simulink library "speedgoatlib_IO682"  (R2024b)
settings: Solver=FixedStepAuto  StartTime=0.0  StopTime=10.0  RelTol=1e-3  EnableMultiTasking=on
undefined symbols (not defined in the file): sg_io682_receive_m_v4, sg_io682_send_m_v4, sg_io682_setup_m_v4, sg_io682_update_scheduled_messages_m_v4, sgarinc429
settings Model: Creator=cschafft  LastModifiedBy=speedgoat\jenkins
settings SolverCC: ConcurrentTasks=on  AlgebraicLoopSolver=TrustRegion  AutoInsertRateTranBlk=on  InsertRTBMode=Never (minimum delay)
settings DataIOCC: LimitDataPoints=on  SaveFormat=StructureWithTime  ReturnWorkspaceOutputs=off
settings OptimizationCC: BlockReduction=off  OptimizeBlockIOStorage=off  BufferReuse=off  ReuseModelBlockBuffer=off  GlobalBufferReuse=off  ExpressionFolding=off  LocalBlockOutputs=off  OptimizeDataStoreBuffers=off  BusAssignmentInplaceUpdate=off
settings DebuggingCC: UnconnectedInputMsg=warning  UnconnectedOutputMsg=warning  UnconnectedLineMsg=warning  AllowSymbolicDim=off  SFUnexpectedBacktrackingDiag=warning  SFNoUnconditionalDefaultTransitionDiag=warning  SFExecutionAtInitializationDiag=none  ArithmeticOperatorsInVariantConditions=warning
settings HardwareCC: ProdBitPerPointer=32  ProdBitPerSizeT=32  ProdBitPerPtrDiffT=32  ProdLargestAtomicFloat=None  ProdWordSize=32  ProdLongLongMode=on  ProdHWDeviceType=Generic->32-bit x86 compatible
settings ModelReferenceCC: EnableRefExpFcnMdlSchedulingChecks=on  PropagateSignalLabelsOutOfModel=off
settings SFSimCC: SimUseLocalCustomCode=off  CustomCodeUndefinedFunction=UseInterfaceOnly
settings RTWCC: Description=Simulink Real-Time  SystemTargetFile=slrt.tlc  TemplateMakefile=slrt_default_tmf  RTWUseLocalCustomCode=off  RTWCompilerOptimization=on  GPUComputeCapability=3.5  DLArmComputeVersion=19.05
settings CodeAppCC: StateflowObjectComments=on
settings SimulinkRealTimeCC: SubcomponentCodeInterfacePackaging=Reusable function  SupportVariableSizeSignals=on  InstructionSetFMA=off  OptimizeReductions=off  LogToMDFFile=off  RL32LogTETModifier=off
settings ConfigComp: CovMetricSettings=dw  CovSaveCumulativeToWorkspaceVar=on  CovSaveSingleToWorkspaceVar=on  CovExternalEMLEnable=off  CovBoundaryAbsTol=1.0e-5

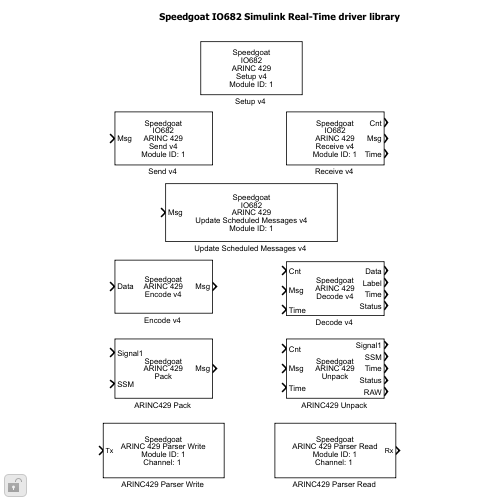
[thumbnail: Simulink's stored preview of the top-level diagram]
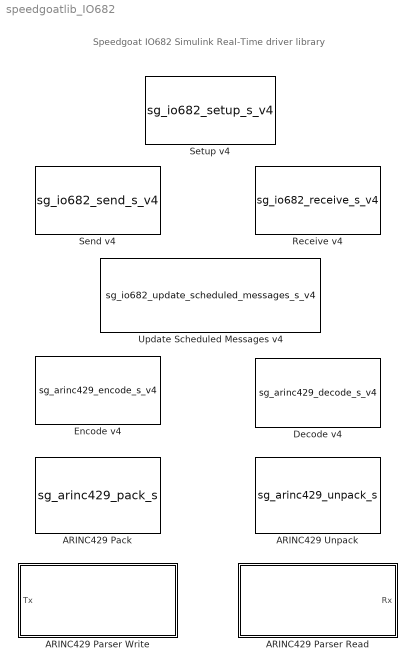
== system speedgoatlib_IO682 ==
  note: Speedgoat IO682 Simulink Real-Time driver library
  "ARINC429 Pack " : S-Function  LoadFcn=sgarinc429.LoadFcnPackUnpack();  FunctionName=sg_arinc429_pack_s  Parameters=sFunParams.decLabel,parSdi,parSsm,sFunParams.signals,sFunParams.hasSsmSig  SFunctionDeploymentMode=off  EnableBusSupport=off  mask(pack_arinc429){parLabel=102, parSdi=0, parSsm=3, parSignals={'Signal1','11','16','BNR','256','0.01','0','-Inf','Inf','off';'SSM','30','2','SSM','1','1','0','-Inf','Inf','off'}}
      mask prompts: parLabel "Label"; parSdi "SDI"; parSsm "SSM"; parSignals "Signals"
      mask help: Speedgoat Driver Block<br>ARINC 429 - Pack<br><br>&copy; 2007 - 2026, Speedgoat GmbH, <a href="matlab: web('www.speedgoat.com','-browser');">www.speedgoat.com</a>
      mask init:
      | sFunParams = sg_arinc429_pack_m.maskInitialization();
      mask Help: eval('sg.utils.help.show(''io_main/refentry_arinc429_pack'');')
      mask DialogControl btnAddSig Prompt: Add Signal
      mask DialogControl btnAddSig Callback: sg_arinc429_pack_m.addSigBtnClb();
      mask DialogControl btnDelSig Prompt: Delete Signal
      mask DialogControl btnDelSig Callback: sg_arinc429_pack_m.delSigBtnClb();
      mask Display: disp('Speedgoat\nARINC 429\nPack');port_label('output',1,'Msg');port_label('input',1,'Signal1');port_label('input',2,'SSM');
  "ARINC429 Parser Read " : Subsystem  mask(read_parser_arinc429){}
      settings: OpenFcn=sgarinc429.OpenFcnRead();
      mask Help: eval('sg.utils.help.show(''io_main/refentry_arinc429_parser_read'');')
      mask Display: disp('Speedgoat\nARINC 429 Parser Read\nModule ID: 1\nChannel: 1 ');
  "ARINC429 Parser Write " : Subsystem  mask(write_parser_arinc429){}
      settings: OpenFcn=sgarinc429.OpenFcnWrite();
      mask Help: eval('sg.utils.help.show(''io_main/refentry_arinc429_parser_write'');')
      mask Display: disp('Speedgoat\nARINC 429 Parser Write\nModule ID: 1\nChannel: 1 ');
  "ARINC429 Unpack " : S-Function  LoadFcn=sgarinc429.LoadFcnPackUnpack();  FunctionName=sg_arinc429_unpack_s  Parameters=sFunParams.decLabel,parSdi,parEnTimeTag,parEnStatus,parEnRaw,sFunParams.signals,sFunParams.hasSsmSig  SFunctionDeploymentMode=off  EnableBusSupport=off  mask(unpack_arinc429){parLabel=102, parSdi=0, parSignals={'Signal1','11','16','BNR','256','0.01','0','-Inf','Inf','off';'SSM','30','2','SSM','1','1','0','-Inf','Inf','off'}, parEnTimeTag=on, parEnStatus=on, parEnRaw=on}
      mask prompts: parLabel "Label"; parSdi "SDI"; parSignals "Signals"; parEnTimeTag "Enable Timestamp Output"; parEnStatus "Enable Status Output"; parEnRaw "Enable RAW Output"
      mask help: Speedgoat Driver Block<br>ARINC 429 - Unpack<br><br>&copy; 2007 - 2026, Speedgoat GmbH, <a href="matlab: web('www.speedgoat.com','-browser');">www.speedgoat.com</a>
      mask init:
      | sFunParams = sg_arinc429_unpack_m.maskInitialization();
      mask Help: eval('sg.utils.help.show(''io_main/refentry_arinc429_unpack'');')
      mask DialogControl btnAddSig Prompt: Add Signal
      mask DialogControl btnAddSig Callback: sg_arinc429_unpack_m.addSigBtnClb();
      mask DialogControl btnDelSig Prompt: Delete Signal
      mask DialogControl btnDelSig Callback: sg_arinc429_unpack_m.delSigBtnClb();
      mask DialogControl Container3 Prompt: Output Ports
      mask Display: disp('Speedgoat\nARINC 429\nUnpack');port_label('input',1,'Cnt');port_label('input',2,'Msg');port_label('input',3,'Time');port_label('output',1,'Signal1');port_label('output',2,'SSM');port_label('output',3,'Time');port_label('output',4,'Status');port_label('output',5,'RAW');
  "Decode v4 " : S-Function  FunctionName=sg_arinc429_decode_s_v4  Parameters=sFunParams.decLabel, sFunParams.dataType, sFunParams.resolution, sFunParams.sdi, parEnSDIBits, parTimeTags, parHoldLastVal, parStatus, parLabelOutput, parSSMOutput  SFunctionDeploymentMode=off  EnableBusSupport=off  mask(decode_arinc429_v4){parLabel=[002], parDataType=BNR, parResolution=[10], parSdi=[0], parEnSDIBits=off, parHoldLastVal=on, parLabelOutput=on, parSSMOutput=off, parTimeTags=on, parStatus=on}
      mask prompts: parLabel "Label (Octal)"; parDataType "Data Type"; parResolution "Scale"; parSdi "SDI"; parEnSDIBits "Use SDI Bits for Data"; parHoldLastVal "Hold Last Value"; parLabelOutput "Enable Label Output"; parSSMOutput "Enable SSM Output"; parTimeTags "Enable Timestamp Output"; parStatus "Enable Status Output"
      mask help: Speedgoat Driver Block<br>ARINC 429 - Decode<br><br>&copy; 2007 - 2026, Speedgoat GmbH, <a href="matlab: web('www.speedgoat.com','-browser');">www.speedgoat.com</a>
      mask init:
      | sFunParams = sg_arinc429_decode_m_v4.runInitializationCommand();
      mask Help: eval('sg.utils.help.show(''io_main/refentry_arinc429_decode_v4'');')
      mask TypeOptions parDataType: RAW | BNR | BCD | Discretes
      mask Callback parDataType: sg_arinc429_decode_m_v4.dataTypeCallback();
      mask Callback parEnSDIBits: sg_arinc429_decode_m_v4.enableSDIBitsCallback();
      mask Display: disp('Speedgoat\nARINC 429\nDecode v4');port_label('input',1,'Cnt');port_label('input',2,'Msg');port_label('input',3,'Time');port_label('output',1,'Data');port_label('output',2,'Label');port_label('output',3,'Time');port_label('output',4,'Status');
  "Encode v4 " : S-Function  FunctionName=sg_arinc429_encode_s_v4  Parameters=sFunParams.decLabel, sFunParams.dataType, sFunParams.resolution, sFunParams.bits, sFunParams.sdi, sFunParams.ssm, parEnSSM, parEnSDIBits  SFunctionDeploymentMode=off  EnableBusSupport=off  mask(encode_arinc429_v4){parLabel=[002], parDataType=BNR, parResolution=[10], parBits=[19], parSdi=[0], parSsm=[3], parEnSDIBits=off, parEnSSM=off}
      mask prompts: parLabel "Label (Octal)"; parDataType "Data Type"; parResolution "Scale"; parBits "Bits to Send"; parSdi "SDI"; parSsm "SSM"; parEnSDIBits "Use SDI Bits for Data"; parEnSSM "Enable SSM Input"
      mask help: Speedgoat Driver Block<br>ARINC 429 - Encode<br><br>&copy; 2007 - 2026, Speedgoat GmbH, <a href="matlab: web('www.speedgoat.com','-browser');">www.speedgoat.com</a>
      mask init:
      | sFunParams = sg_arinc429_encode_m_v4.runInitializationCommand();
      mask Help: eval('sg.utils.help.show(''io_main/refentry_arinc429_encode_v4'');')
      mask TypeOptions parDataType: RAW | BNR | BCD | Discretes
      mask Callback parDataType: sg_arinc429_encode_m_v4.dataTypeCallback();
      mask Callback parEnSDIBits: sg_arinc429_encode_m_v4.enableSDIBitsCallback();
      mask Callback parEnSSM: sg_arinc429_encode_m_v4.enableSSMCallback();
      mask Display: disp('Speedgoat\nARINC 429\nEncode v4');port_label('output',1,'Msg');port_label('input',1,'Data');
  "Receive v4 " : S-Function  InitFcn=sg_io682_receive_m_v4.runInitFcn();  FunctionName=sg_io682_receive_s_v4  Parameters=parModuleId, parChannel, parMaxWords, parSampleTime, parEnTimeTags  SFunctionDeploymentMode=off  EnableBusSupport=off  mask(receive_IO682_v4){parModuleId=1, parChannel=1, parMaxWords=50, parSampleTime=-1, parEnTimeTags=on}
      mask prompts: parModuleId "Module ID"; parChannel "Channel"; parMaxWords "Max Number of Messages to Return"; parSampleTime "Sample Time [s]"; parEnTimeTags "Provide Timestamps"
      mask help: Speedgoat Driver Block<br>IO682 - Receive<br><br>&copy; 2007 - 2026, Speedgoat GmbH, <a href="matlab: web('www.speedgoat.com','-browser');">www.speedgoat.com</a>
      mask init:
      | sg_io682_receive_m_v4.runMaskInitialization();
      mask Help: eval('sg.utils.help.show(''io_main/refentry_io682_receive_v4'');')
      mask TypeOptions parChannel: 1 | 2 | 3 | 4 | 5 | 6 | 7 | 8 | 9 | 10 | 11 | 12 | 13 | 14 | 15 | 16
      mask Display: disp('Speedgoat\nIO682\nARINC 429\nReceive v4\nModule ID: 1');port_label('output',1,'Cnt');port_label('output',2,'Msg');port_label('output',3,'Time');
  "Send v4 " : S-Function  InitFcn=sg_io682_send_m_v4.runInitFcn();  FunctionName=sg_io682_send_s_v4  Parameters=parModuleId, parChannel, parSampleTime, parTxCtrl  SFunctionDeploymentMode=off  EnableBusSupport=off  mask(send_IO682_v4){parModuleId=1, parChannel=1, parSampleTime=-1, parTxCtrl=off}
      mask prompts: parModuleId "Module ID"; parChannel "Channel"; parSampleTime "Sample Time [s]"; parTxCtrl "Show Transmission Control Input"
      mask help: Speedgoat Driver Block<br>IO682 - Send<br><br>&copy; 2007 - 2026, Speedgoat GmbH, <a href="matlab: web('www.speedgoat.com','-browser');">www.speedgoat.com</a>
      mask init:
      | sg_io682_send_m_v4.runMaskInitialization();
      mask Help: eval('sg.utils.help.show(''io_main/refentry_io682_send_v4'');')
      mask TypeOptions parChannel: 1 | 2 | 3 | 4 | 5 | 6 | 7 | 8 | 9 | 10 | 11 | 12 | 13 | 14 | 15 | 16
      mask Display: disp('Speedgoat\nIO682\nARINC 429\nSend v4\nModule ID: 1');port_label('input',1,'Msg');
  "Setup v4 " : S-Function  InitFcn=sg_io682_setup_m_v4.runInitFcn();  FunctionName=sg_io682_setup_s_v4  Parameters=parModuleId, parBoardVariant, parPciSlot, parHwDeviceId, parScheduledMessages, parChInConfig,parChOutConfig  SFunctionModules=sg_io682_v4  SFunctionDeploymentMode=off  EnableBusSupport=off  mask(setup_IO682_v4){parModuleId=1, parBoardVariant=IO682-2-2, parPciSlot=-1, parChannelMode=Manual, parInBitRate1=100000, parInBufferMode1=Individual, parInEnable1=on, parInParity1=on, parInInternalWrap1=off, parInBitRate2=100000, parInBufferMode2=Individual, parInEnable2=on, parInParity2=on, parInInternalWrap2=off, parInBitRate3=100000, parInBufferMode3=Individual, parInEnable3=on, parInParity3=on, parInInternalWrap3=off, parInBitRate4=100000, parInBufferMode4=Individual, parInEnable4=on, parInParity4=on, parInInternalWrap4=off, parInBitRate5=100000, parInBufferMode5=Individual, parInEnable5=on, parInParity5=on, parInInternalWrap5=off, parInBitRate6=100000, parInBufferMode6=Individual, parInEnable6=on, parInParity6=on, parInInternalWrap6=off, parInBitRate7=100000, parInBufferMode7=Individual, parInEnable7=on, parInParity7=on, parInInternalWrap7=off, parInBitRate8=100000, parInBufferMode8=Individual, parInEnable8=on, parInParity8=on, parInInternalWrap8=off, parInBitRate9=100000, parInBufferMode9=Individual, parInEnable9=on, parInParity9=on, parInInternalWrap9=off, parInBitRate10=100000, parInBufferMode10=Individual, parInEnable10=on, parInParity10=on, parInInternalWrap10=off, parInBitRate11=100000, parInBufferMode11=Individual, parInEnable11=on, parInParity11=on, parInInternalWrap11=off, parInBitRate12=100000, parInBufferMode12=Individual, parInEnable12=on, parInParity12=on, parInInternalWrap12=off, parInBitRate13=100000, parInBufferMode13=Individual, parInEnable13=on, parInParity13=on, parInInternalWrap13=off, parInBitRate14=100000, parInBufferMode14=Individual, parInEnable14=on, parInParity14=on, parInInternalWrap14=off, parInBitRate15=100000, parInBufferMode15=Individual, parInEnable15=on, parInParity15=on, parInInternalWrap15=off, parInBitRate16=100000, parInBufferMode16=Individual, parInEnable16=on, parInParity16=on, parInInternalWrap16=off, parOutBitRate1=100000, parOutParity1=Odd, parOutProtocolError1=None, parOutEnable1=on, parOutBitRate2=100000, parOutParity2=Odd, parOutProtocolError2=None, parOutEnable2=on, parOutBitRate3=100000, parOutParity3=Odd, parOutProtocolError3=None, parOutEnable3=on, parOutBitRate4=100000, parOutParity4=Odd, parOutProtocolError4=None, parOutEnable4=on, parOutBitRate5=100000, parOutParity5=Odd, parOutProtocolError5=None, parOutEnable5=on, parOutBitRate6=100000, parOutParity6=Odd, parOutProtocolError6=None, parOutEnable6=on, parOutBitRate7=100000, parOutParity7=Odd, parOutProtocolError7=None, parOutEnable7=on, parOutBitRate8=100000, parOutParity8=Odd, parOutProtocolError8=None, parOutEnable8=on, parOutBitRate9=100000, parOutParity9=Odd, parOutProtocolError9=None, parOutEnable9=on, parOutBitRate10=100000, parOutParity10=Odd, parOutProtocolError10=None, parOutEnable10=on, parOutBitRate11=100000, parOutParity11=Odd, parOutProtocolError11=None, parOutEnable11=on, parOutBitRate12=100000, parOutParity12=Odd, parOutProtocolError12=None, parOutEnable12=on, parOutBitRate13=100000, parOutParity13=Odd, parOutProtocolError13=None, parOutEnable13=on, parOutBitRate14=100000, parOutParity14=Odd, parOutProtocolError14=None, parOutEnable14=on, parOutBitRate15=100000, parOutParity15=Odd, parOutProtocolError15=None, parOutEnable15=on, parOutBitRate16=100000, parOutParity16=Odd, parOutProtocolError16=None, parOutEnable16=on, parChConfigFile='', parScheduleMode=Manual, parScheduledMsgConfigFile='', parHwDeviceId=hex2dec('0830'), parChInConfig=[158 8 7 7 1;158 8 7 7 1], parChOutConfig=[158 0 4 7;158 0 4 7], parScheduledMessages=0}
      mask prompts: parModuleId "Module ID"; parBoardVariant "IO682 Variant"; parPciSlot "PCI Slot (-1: autosearch)"; parChannelMode "Mode"; parInBitRate1 "Bit Rate"; parInBufferMode1 "Buffer Mode"; parInEnable1 "Enable"; parInParity1 "Parity Check"; parInInternalWrap1 "Internal Wrap"; parInBitRate2 "Bit Rate"; parInBufferMode2 "Buffer Mode"; parInEnable2 "Enable"; parInParity2 "Parity Check"; parInInternalWrap2 "Internal Wrap"; parInBitRate3 "Bit Rate"; parInBufferMode3 "Buffer Mode"; parInEnable3 "Enable"; parInParity3 "Parity Check"; parInInternalWrap3 "Internal Wrap"; parInBitRate4 "Bit Rate"; parInBufferMode4 "Buffer Mode"; parInEnable4 "Enable"; parInParity4 "Parity Check"; parInInternalWrap4 "Internal Wrap"; parInBitRate5 "Bit Rate"; parInBufferMode5 "Buffer Mode"; parInEnable5 "Enable"; parInParity5 "Parity Check"; parInInternalWrap5 "Internal Wrap"; parInBitRate6 "Bit Rate"; parInBufferMode6 "Buffer Mode"; parInEnable6 "Enable"; parInParity6 "Parity Check"; parInInternalWrap6 "Internal Wrap"; parInBitRate7 "Bit Rate"; parInBufferMode7 "Buffer Mode"; parInEnable7 "Enable"; parInParity7 "Parity Check"; parInInternalWrap7 "Internal Wrap"; parInBitRate8 "Bit Rate"; parInBufferMode8 "Buffer Mode"; parInEnable8 "Enable"; parInParity8 "Parity Check"; parInInternalWrap8 "Internal Wrap"; parInBitRate9 "Bit Rate"; parInBufferMode9 "Buffer Mode"; parInEnable9 "Enable"; parInParity9 "Parity Check"; parInInternalWrap9 "Internal Wrap"; parInBitRate10 "Bit Rate"; parInBufferMode10 "Buffer Mode"; parInEnable10 "Enable"; parInParity10 "Parity Check"; parInInternalWrap10 "Internal Wrap"; parInBitRate11 "Bit Rate"; parInBufferMode11 "Buffer Mode"; parInEnable11 "Enable"; parInParity11 "Parity Check"; parInInternalWrap11 "Internal Wrap"; parInBitRate12 "Bit Rate"; parInBufferMode12 "Buffer Mode"; parInEnable12 "Enable"; parInParity12 "Parity Check"; parInInternalWrap12 "Internal Wrap"; parInBitRate13 "Bit Rate"; parInBufferMode13 "Buffer Mode"; parInEnable13 "Enable"; parInParity13 "Parity Check"; parInInternalWrap13 "Internal Wrap"; parInBitRate14 "Bit Rate"; parInBufferMode14 "Buffer Mode"; parInEnable14 "Enable"; parInParity14 "Parity Check"; parInInternalWrap14 "Internal Wrap"; parInBitRate15 "Bit Rate"; parInBufferMode15 "Buffer Mode"; parInEnable15 "Enable"; parInParity15 "Parity Check"; parInInternalWrap15 "Internal Wrap"; parInBitRate16 "Bit Rate"; parInBufferMode16 "Buffer Mode"; parInEnable16 "Enable"; parInParity16 "Parity Check"; parInInternalWrap16 "Internal Wrap"; parOutBitRate1 "Bit Rate"; parOutParity1 "Parity"; parOutProtocolError1 "Protocol Error"; parOutEnable1 "Enable"; parOutBitRate2 "Bit Rate"; parOutParity2 "Parity"; parOutProtocolError2 "Protocol Error"; parOutEnable2 "Enable"; parOutBitRate3 "Bit Rate"; parOutParity3 "Parity"; parOutProtocolError3 "Protocol Error"; parOutEnable3 "Enable"; parOutBitRate4 "Bit Rate"; parOutParity4 "Parity"; parOutProtocolError4 "Protocol Error"; parOutEnable4 "Enable"; parOutBitRate5 "Bit Rate"; parOutParity5 "Parity"; parOutProtocolError5 "Protocol Error"; parOutEnable5 "Enable"; parOutBitRate6 "Bit Rate"; parOutParity6 "Parity"; parOutProtocolError6 "Protocol Error"; parOutEnable6 "Enable"; parOutBitRate7 "Bit Rate"; parOutParity7 "Parity"; parOutProtocolError7 "Protocol Error"; parOutEnable7 "Enable"; parOutBitRate8 "Bit Rate"; parOutParity8 "Parity"; parOutProtocolError8 "Protocol Error"; parOutEnable8 "Enable"; parOutBitRate9 "Bit Rate"; parOutParity9 "Parity"; parOutProtocolError9 "Protocol Error"; parOutEnable9 "Enable"; parOutBitRate10 "Bit Rate"; parOutParity10 "Parity"; parOutProtocolError10 "Protocol Error"; parOutEnable10 "Enable"; parOutBitRate11 "Bit Rate"; parOutParity11 "Parity"; parOutProtocolError11 "Protocol Error"; parOutEnable11 "Enable"; parOutBitRate12 "Bit Rate"; parOutParity12 "Parity"; parOutProtocolError12 "Protocol Error"; parOutEnable12 "Enable"; parOutBitRate13 "Bit Rate"; parOutParity13 "Parity"; parOutProtocolError13 "Protocol Error"; parOutEnable13 "Enable"; parOutBitRate14 "Bit Rate"; parOutParity14 "Parity"; parOutProtocolError14 "Protocol Error"; parOutEnable14 "Enable"; parOutBitRate15 "Bit Rate"; parOutParity15 "Parity"; parOutProtocolError15 "Protocol Error"; parOutEnable15 "Enable"; parOutBitRate16 "Bit Rate"; parOutParity16 "Parity"; parOutProtocolError16 "Protocol Error"; parOutEnable16 "Enable"; parChConfigFile "Channels Configuration File"; parScheduleMode "Mode"; parScheduledMsgConfigFile "Scheduled Messages Configuration File"; parChInConfig "In Ch Config List"; parChOutConfig "Out Ch Config List"; parScheduledMessages "Message List"
      mask help: Speedgoat Driver Block<br>IO682 - Setup<br><br>&copy; 2007 - 2026, Speedgoat GmbH, <a href="matlab: web('www.speedgoat.com','-browser');">www.speedgoat.com</a>
      mask init:
      | sg_io682_setup_m_v4.runMaskInitialization();
      mask Help: eval('sg.utils.help.show(''io_main/refentry_io682_setup_v4'');')
      mask TypeOptions parBoardVariant: IO682-2-2 | IO682-4-4 | IO682-8-8 | IO682-16-16
      mask Callback parBoardVariant: sg_io682_setup_m_v4.runBoardVariantCb();
      mask TypeOptions parChannelMode: Manual | Configuration File
      mask Callback parChannelMode: sg_io682_setup_m_v4.runChannelModeCb();
      mask TypeOptions parInBufferMode1: Individual | Merged
      mask TypeOptions parInBufferMode2: Individual | Merged
      mask TypeOptions parInBufferMode3: Individual | Merged
      mask TypeOptions parInBufferMode4: Individual | Merged
      mask TypeOptions parInBufferMode5: Individual | Merged
      mask TypeOptions parInBufferMode6: Individual | Merged
      mask TypeOptions parInBufferMode7: Individual | Merged
      mask TypeOptions parInBufferMode8: Individual | Merged
      mask TypeOptions parInBufferMode9: Individual | Merged
      mask TypeOptions parInBufferMode10: Individual | Merged
      mask TypeOptions parInBufferMode11: Individual | Merged
      mask TypeOptions parInBufferMode12: Individual | Merged
      mask TypeOptions parInBufferMode13: Individual | Merged
      mask TypeOptions parInBufferMode14: Individual | Merged
      mask TypeOptions parInBufferMode15: Individual | Merged
      mask TypeOptions parInBufferMode16: Individual | Merged
      mask TypeOptions parOutParity1: None | Odd | Even
      mask TypeOptions parOutProtocolError1: None | Bit Count High | Bit Count Low | Short Gap
      mask TypeOptions parOutParity2: None | Odd | Even
      mask TypeOptions parOutProtocolError2: None | Bit Count High | Bit Count Low | Short Gap
      mask TypeOptions parOutParity3: None | Odd | Even
      mask TypeOptions parOutProtocolError3: None | Bit Count High | Bit Count Low | Short Gap
      mask TypeOptions parOutParity4: None | Odd | Even
      mask TypeOptions parOutProtocolError4: None | Bit Count High | Bit Count Low | Short Gap
      mask TypeOptions parOutParity5: None | Odd | Even
      mask TypeOptions parOutProtocolError5: None | Bit Count High | Bit Count Low | Short Gap
      mask TypeOptions parOutParity6: None | Odd | Even
      mask TypeOptions parOutProtocolError6: None | Bit Count High | Bit Count Low | Short Gap
      mask TypeOptions parOutParity7: None | Odd | Even
      mask TypeOptions parOutProtocolError7: None | Bit Count High | Bit Count Low | Short Gap
      mask TypeOptions parOutParity8: None | Odd | Even
      mask TypeOptions parOutProtocolError8: None | Bit Count High | Bit Count Low | Short Gap
      mask TypeOptions parOutParity9: None | Odd | Even
      mask TypeOptions parOutProtocolError9: None | Bit Count High | Bit Count Low | Short Gap
      mask TypeOptions parOutParity10: None | Odd | Even
      mask TypeOptions parOutProtocolError10: None | Bit Count High | Bit Count Low | Short Gap
      mask TypeOptions parOutParity11: None | Odd | Even
      mask TypeOptions parOutProtocolError11: None | Bit Count High | Bit Count Low | Short Gap
      mask TypeOptions parOutParity12: None | Odd | Even
      mask TypeOptions parOutProtocolError12: None | Bit Count High | Bit Count Low | Short Gap
      mask TypeOptions parOutParity13: None | Odd | Even
      mask TypeOptions parOutProtocolError13: None | Bit Count High | Bit Count Low | Short Gap
      mask TypeOptions parOutParity14: None | Odd | Even
      mask TypeOptions parOutProtocolError14: None | Bit Count High | Bit Count Low | Short Gap
      mask TypeOptions parOutParity15: None | Odd | Even
      mask TypeOptions parOutProtocolError15: None | Bit Count High | Bit Count Low | Short Gap
      mask TypeOptions parOutParity16: None | Odd | Even
      mask TypeOptions parOutProtocolError16: None | Bit Count High | Bit Count Low | Short Gap
      mask TypeOptions parScheduleMode: Manual | Configuration File
      mask Callback parScheduleMode: sg_io682_setup_m_v4.runScheduleModeCb();
      mask DialogControl tabMain Prompt: Main
      mask DialogControl boxModuleSettings Prompt: Module Settings
      mask DialogControl tabChannelConfig Prompt: Channel Configuration
      mask DialogControl boxInputChannelConfig Prompt: Input Channels
      mask DialogControl parInChannel1 Prompt: Channel 01:
      mask DialogControl parInChannel2 Prompt: Channel 02:
      mask DialogControl parInChannel3 Prompt: Channel 03:
      mask DialogControl parInChannel4 Prompt: Channel 04:
      mask DialogControl parInChannel5 Prompt: Channel 05:
      mask DialogControl parInChannel6 Prompt: Channel 06:
      mask DialogControl parInChannel7 Prompt: Channel 07:
      mask DialogControl parInChannel8 Prompt: Channel 08:
      mask DialogControl parInChannel9 Prompt: Channel 09:
      mask DialogControl parInChannel10 Prompt: Channel 10:
      mask DialogControl parInChannel11 Prompt: Channel 11:
      mask DialogControl parInChannel12 Prompt: Channel 12:
      mask DialogControl parInChannel13 Prompt: Channel 13:
      mask DialogControl parInChannel14 Prompt: Channel 14:
      mask DialogControl parInChannel15 Prompt: Channel 15:
      mask DialogControl parInChannel16 Prompt: Channel 16:
      mask DialogControl boxOutputChannelConfig Prompt: Output Channels
      mask DialogControl parOutChannel1 Prompt: Channel 01:
      mask DialogControl parOutChannel2 Prompt: Channel 02:
      mask DialogControl parOutChannel3 Prompt: Channel 03:
      mask DialogControl parOutChannel4 Prompt: Channel 04:
      mask DialogControl parOutChannel5 Prompt: Channel 05:
      mask DialogControl parOutChannel6 Prompt: Channel 06:
      mask DialogControl parOutChannel7 Prompt: Channel 07:
      mask DialogControl parOutChannel8 Prompt: Channel 08:
      mask DialogControl parOutChannel9 Prompt: Channel 09:
      mask DialogControl parOutChannel10 Prompt: Channel 10:
      mask DialogControl parOutChannel11 Prompt: Channel 11:
      mask DialogControl parOutChannel12 Prompt: Channel 12:
      mask DialogControl parOutChannel13 Prompt: Channel 13:
      mask DialogControl parOutChannel14 Prompt: Channel 14:
      mask DialogControl parOutChannel15 Prompt: Channel 15:
      mask DialogControl parOutChannel16 Prompt: Channel 16:
      mask DialogControl Container23 Prompt: Configuration File
      mask DialogControl btnChBrowse Prompt: Browse
      mask DialogControl btnChBrowse Callback: sg_io682_setup_m_v4.runChannelBrowseCb();
      mask DialogControl btnChRefresh Prompt: Refresh Data
      mask DialogControl btnChRefresh Callback: sg_io682_setup_m_v4.runChannelRefreshCb();
      mask DialogControl btnChSave Prompt: Save Configuration
      mask DialogControl btnChSave Callback: sg_io682_setup_m_v4.runChannelSaveCb();
      mask DialogControl Container11 Prompt: Scheduled Messages
      mask DialogControl boxScheduleMsg Prompt: Schedule Messages
      mask DialogControl btnScheduleMsg Prompt: Create Message List
      mask DialogControl btnScheduleMsg Callback: sg_io682_setup_m_v4.runScheduleMsgCb();
      mask DialogControl Container27 Prompt: Configuration File
      mask DialogControl btnScheduleBrowse Prompt: Browse
      mask DialogControl btnScheduleBrowse Callback: sg_io682_setup_m_v4.runScheduleBrowseCb();
      mask DialogControl btnScheduleRefresh Prompt: Refresh Data
      mask DialogControl btnScheduleRefresh Callback: sg_io682_setup_m_v4.runScheduleRefreshCb();
      mask DialogControl btnScheduleSave Prompt: Save Configuration
      mask DialogControl btnScheduleSave Callback: sg_io682_setup_m_v4.runScheduleSaveCb();
      mask Display: disp('Speedgoat\nIO682\nARINC 429\nSetup v4\nModule ID: 1');
  "Update Scheduled Messages v4 " : S-Function  InitFcn=sg_io682_update_scheduled_messages_m_v4.runInitFcn();  FunctionName=sg_io682_update_scheduled_messages_s_v4  Parameters=parModuleId, parMessageId, parSampleTime, parEnRate  SFunctionDeploymentMode=off  EnableBusSupport=off  mask(update_scheduled_messages_IO682_v4){parModuleId=1, parMessageId=1, parSampleTime=-1, parEnRate=off}
      mask prompts: parModuleId "Module ID"; parMessageId "Message Index"; parSampleTime "Sample Time [s]"; parEnRate "Show Rate Input"
      mask help: Speedgoat Driver Block<br>IO682 - Update Scheduled Messages<br><br>&copy; 2007 - 2026, Speedgoat GmbH, <a href="matlab: web('www.speedgoat.com','-browser');">www.speedgoat.com</a>
      mask init:
      | sg_io682_update_scheduled_messages_m_v4.runMaskInitialization();
      mask Help: eval('sg.utils.help.show(''io_main/refentry_io682_update_scheduled_messages_v4'');')
      mask Display: disp('Speedgoat\nIO682\nARINC 429\nUpdate Scheduled Messages v4\nModule ID: 1');port_label('input',1,'Msg');

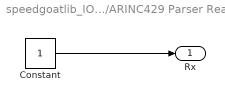
== system speedgoatlib_IO682/ARINC429 Parser Read  ==
  Constant : Constant
  Rx : Outport
  wires:
  Constant/1 -> Rx/1

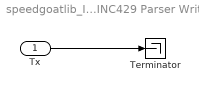
== system speedgoatlib_IO682/ARINC429 Parser Write  ==
  Tx : Inport
  Terminator : Terminator
  wires:
  Tx/1 -> Terminator/1
